simulink model "Wireless_charging"  (R2024a)
settings: Solver=VariableStepAuto  StartTime=0.0  StopTime=1  RelTol=1e-3
undefined symbols (not defined in the file): Ion, Lithium
libraries: spsSeriesRLCBranchLib x5, spsDiodeLib x4, spsMultimeterLib x4, spsIGBTDiodeLib x4, spsMeanLib x4, spsCurrentMeasurementLib x2, spsVoltageMeasurementLib x2, spsACVoltageSourceLib x1, spsUniversalBridgeLib x1, spsPWMGeneratorDCDCLib x1, spsBatteryLib x1, spsMutualInductanceLib x1
settings Model: Creator=User  LastModifiedBy=User

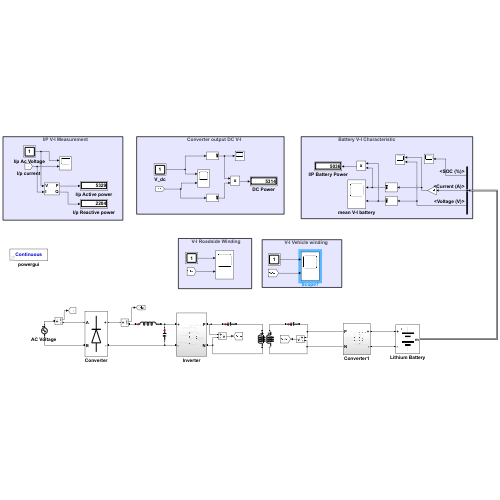
[thumbnail: Simulink's stored preview of the top-level diagram]
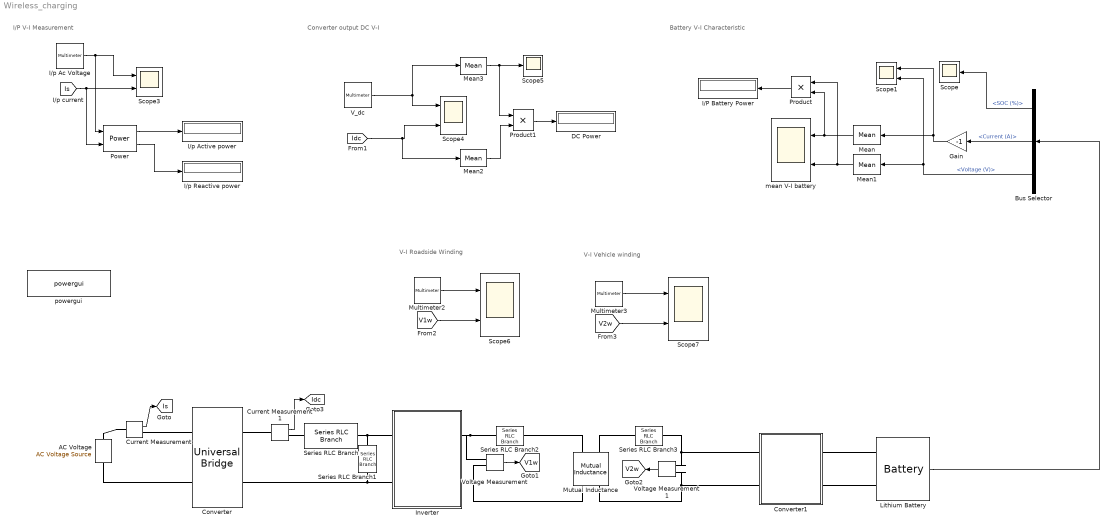
== system Wireless_charging ==
  note: V-I Roadside Winding
  note: V-I Vehicle winding
  note: Battery V-I Characteristic
  note: I/P V-I Measurement
  note: Converter output DC V-I
  "AC Voltage " : spsACVoltageSourceLib/AC Voltage Source  Amplitude=325  Phase=0  Frequency=50  SampleTime=0  Measurements=Voltage  BusType=swing  Pref=10e3  Qref=0  Qmin=-inf  Qmax=+inf
  Bus Selector : BusSelector  OutputSignals=SOC (%),Current (A),Voltage (V)
  Converter : spsUniversalBridgeLib/Universal Bridge  Arms=2  SnubberResistance=1e5  SnubberCapacitance=inf  Device=Diodes  Ron=1e-3  Lon=0  ForwardVoltages="[  0  0  ]"  ForwardVoltage=0  GTOparameters=[ 10e-6 , 20e-6 ]  IGBTparameters=[ 1e-6 , 2e-6 ]  Measurements=All voltages and currents  Measurements_2=None  converterType=Rectifier
  Converter1 : Subsystem
  Current Measurement : spsCurrentMeasurementLib/Current Measurement  PhasorSimulation=off  OutputType=Complex  PSBequivalent=0
  Current Measurement1 : spsCurrentMeasurementLib/Current Measurement  PhasorSimulation=off  OutputType=Complex  PSBequivalent=0
  DC Power : Display
  Gain : Gain  Gain=-1
  I/P Battery Power : Display
  I/p Ac Voltage : spsMultimeterLib/Multimeter  L=15  sel=8  yselected={}  Gain=1  OutputType=Complex  PlotAtSimulationStop=off  PhasorSimulation=off
  I/p Active power : Display
  I/p Reactive power : Display
  Inverter : Subsystem
  Lithium Battery : spsBatteryLib/Battery  BatType=Lithium-Ion  ShowTempParam=off  ThermalPreset=no  ShowAgeParam=off  NomV=360  NomQ=100  SOC=50  Batt_Tr=1  PresetModel=on  MaxQ=100  MinV=270  FullV=419.0354  Dis_rate=43.4783  R=0.036  Normal_OP=90.4348  expZone="[388.9389      4.913043]"  current=[6.5 13 32.5]  Units=Time  Tci=20  NomT=20  T2=-30  MaxQ2=4.8  FullV2=7.1  Normal_OP2=5.655  expZone2="[6.58           1]"  Rca=0.6  ti=2000  Dp=0  Neq0=0  Tsim=1e6  Ta1=25  Qeol=5.4*0.9  Reol=0.013333*1.2  Char_age=[2.3478, 3]  Dis_age=[2.3478, 10]  N1=1500  N2=10500  N3=1000  N4=1400  Ta2=45  N5=950
  Mean{,1..3} (4 alike) : spsMeanLib/Mean  Freq=50  Vinit=0  Ts=0
  Multimeter2 : spsMultimeterLib/Multimeter  L=15  sel=10  yselected={}  Gain=1  OutputType=Complex  PlotAtSimulationStop=off  PhasorSimulation=off
  Multimeter3 : spsMultimeterLib/Multimeter  L=15  sel=11  yselected={}  Gain=1  OutputType=Complex  PlotAtSimulationStop=off  PhasorSimulation=off
  Mutual Inductance : spsMutualInductanceLib/Mutual Inductance  LConnTagsString=a|b  RConnTagsString=A|B  TypeOfMutual=Two or three windings with equal mutual terms  NumberOfWindings=3  SelfImpedance1=[1e-3 266.16e-06]  SelfImpedance2=[ 1e-3 266.16e-06]  ThreeWindings=off  SelfImpedance3=[ 1.1 1.1e-03]  MutualImpedance=[0 85.46e-06]  InductanceMatrix="[1.0 0.9  0.9 ;  0.9 1.0  0.9;  0.9 0.9 1.0 ] * 1e-3"  ResistanceMatrix="[1.0 0.9  0.9 ;  0.9 1.0  0.9;  0.9 0.9 1.0 ]"  Measurements=None
      settings: LibrarySourceBlock=sps_lib/Passives/Mutual Inductance
  Power : spsPowerLib/Power  Freq=50  Vinit=[1, 0]  Iinit=[1, 0]  Ts=0
  Product : Product
  Product1 : Product
  Scope : Scope
  Scope{1,3..4,6..7} (5 alike) : Scope  NumInputPorts=2
  Scope5 : Scope
  Series RLC Branch : spsSeriesRLCBranchLib/Series RLC Branch  LConnTagsString=__new0  RConnTagsString=__new0  BranchType=L  Resistance=1  Inductance=10e-3  SetiL0=off  InitialCurrent=0  Capacitance=1e-6  Setx0=off  InitialVoltage=0  Measurements=Branch current
  Series RLC Branch1 : spsSeriesRLCBranchLib/Series RLC Branch  LConnTagsString=__new0  RConnTagsString=__new0  BranchType=C  Resistance=1  Inductance=1e-3  SetiL0=off  InitialCurrent=0  Capacitance=300e-6  Setx0=off  InitialVoltage=0  Measurements=None
  Series RLC Branch2 : spsSeriesRLCBranchLib/Series RLC Branch  LConnTagsString=__new0  RConnTagsString=__new0  BranchType=C  Resistance=1  Inductance=1e-3  SetiL0=off  InitialCurrent=0  Capacitance=105.74e-9  Setx0=off  InitialVoltage=0  Measurements=Branch current
  Series RLC Branch3 : spsSeriesRLCBranchLib/Series RLC Branch  LConnTagsString=__new0  RConnTagsString=__new0  BranchType=C  Resistance=1  Inductance=1e-3  SetiL0=off  InitialCurrent=0  Capacitance=109.634e-9  Setx0=off  InitialVoltage=0  Measurements=Branch current
  V_dc : spsMultimeterLib/Multimeter  L=15  sel=7  yselected={}  Gain=1  OutputType=Complex  PlotAtSimulationStop=off  PhasorSimulation=off
  Voltage Measurement : spsVoltageMeasurementLib/Voltage Measurement  PhasorSimulation=off  OutputType=Complex  PSBequivalent=0
  Voltage Measurement1 : spsVoltageMeasurementLib/Voltage Measurement  PhasorSimulation=off  OutputType=Complex  PSBequivalent=0
  mean V-I battery : Scope  NumInputPorts=2
  powergui : sps_lib/powergui  Priority=1  SimulationMode=Continuous  SampleTime=50e-6  frequency=60  Iterations=50  frequencyindice=50  Pbase=100e6  ErrMax=1e-4  UnitsV=kV  UnitsW=MW  buscounter=0  FunctionMessages=off  echomessages=off  EnableUseOfTLC=off  CurrentSourceSwitches=off  DisableSnubberDevices=off  DisableRonSwitches=off  DisableVfSwitches=off  DisplayEquations=off  AutomaticDiscreteSolvers=off  SolverType=Tustin/Backward Euler (TBE)  Interpol=off  ExternalGateDelay=off  methode=off  Ts=100  x0status=blocks  SPID=on  SwTol=0  HookPort=off  NonlinearTolerance=1e-4  nMaxIteration=100  ContinueOnMaxIteration=off  RestoreLinks=warning  ResistiveCurrentMeasurement=off  Frange=[0:2:500]  Ylog=off  Xlog=on  ShowGrid=off  save=off  variable=ZData  structure=0  ZoomFFT=off  StartTime=0.0  cycles=1  DisplayStyle=1  fundamental=60  FreqAxis=off  MaxFrequency=1000  frequencyindicesteady=1  RmsSteady=1  display=off
  tag scope: Idc=global, Is=global, V1w=global, V2w=global
  wires:
  Current Measurement/1 -> [Is]
  Voltage Measurement/1 -> [V1w]
  Voltage Measurement1/1 -> [V2w]
  Lithium Battery/1 -> Bus Selector/1
  Bus Selector/1 -> Scope/1  "<SOC (%)>"
  Bus Selector/2 -> Gain/1  "<Current (A)>"
  Gain/1 -> Mean/1, Scope1/1
  Bus Selector/3 -> Mean1/1, Scope1/2  "<Voltage (V)>"
  Mean/1 -> Product/2, mean V-I battery/1
  Mean1/1 -> Product/1, mean V-I battery/2
  Product/1 -> I/P Battery Power/1
  I/p Ac Voltage/1 -> Scope3/1, Power/1
  [Is] -> Power/2, Scope3/2
  Current Measurement1/1 -> [Idc]
  Power/2 -> I/p Reactive power/1
  Power/1 -> I/p Active power/1
  V_dc/1 -> Scope4/1, Mean3/1
  [Idc] -> Mean2/1, Scope4/2
  Mean3/1 -> Product1/1, Scope5/1
  Mean2/1 -> Product1/2
  Product1/1 -> DC Power/1
  Multimeter2/1 -> Scope6/1
  [V1w] -> Scope6/2
  Multimeter3/1 -> Scope7/1
  [V2w] -> Scope7/2
  connections:
  Current Measurement/LConn1 -- "AC Voltage "/RConn1
  Current Measurement/RConn1 -- Converter/LConn1
  Current Measurement1/LConn1 -- Converter/RConn1
  Series RLC Branch/RConn1 -- Inverter/LConn1 -- Series RLC Branch1/LConn1
  Current Measurement1/RConn1 -- Series RLC Branch/LConn1
  "AC Voltage "/LConn1 -- Converter/LConn2
  Converter/RConn2 -- Inverter/LConn2 -- Series RLC Branch1/RConn1
  Inverter/RConn1 -- Series RLC Branch2/LConn1 -- Voltage Measurement/LConn1
  Inverter/RConn2 -- Voltage Measurement/LConn2 -- Mutual Inductance/RConn1
  Series RLC Branch2/RConn1 -- Mutual Inductance/LConn1
  Series RLC Branch3/LConn1 -- Mutual Inductance/LConn2
  Voltage Measurement1/LConn1 -- Series RLC Branch3/RConn1 -- Converter1/LConn1
  Voltage Measurement1/LConn2 -- Mutual Inductance/RConn2 -- Converter1/LConn2
  Lithium Battery/LConn1 -- Converter1/RConn1
  Lithium Battery/LConn2 -- Converter1/RConn2

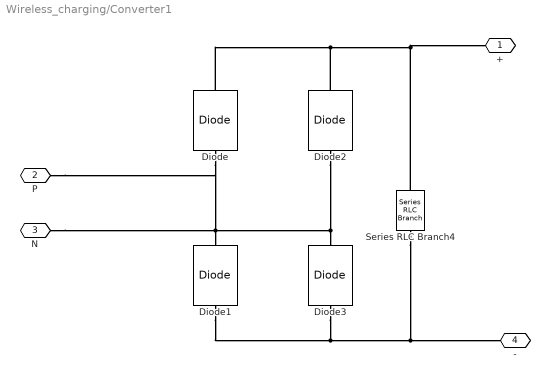
== system Wireless_charging/Converter1 ==
  Diode{,1..3} (4 alike) : spsDiodeLib/Diode  Ron=0.001  Lon=0  Vf=0.8  IC=0  UseSnubber=0  Rs=500  Cs=250e-9  Measurements=off
  Series RLC Branch4 : spsSeriesRLCBranchLib/Series RLC Branch  LConnTagsString=__new0  RConnTagsString=__new0  BranchType=C  Resistance=1  Inductance=1e-3  SetiL0=off  InitialCurrent=0  Capacitance=300e-06  Setx0=off  InitialVoltage=0  Measurements=Branch voltage
  + : PMIOPort  Side=Right
  P : PMIOPort  Port=2  Side=Left
  N : PMIOPort  Port=3  Side=Left
  - : PMIOPort  Port=4  Side=Right
  connections:
  Diode1/LConn1 -- Diode3/LConn1 -- -/RConn1 -- Series RLC Branch4/RConn1
  Diode1/RConn1 -- P/RConn1 -- Diode/LConn1
  Diode3/RConn1 -- N/RConn1 -- Diode2/LConn1
  Diode/RConn1 -- Diode2/RConn1 -- +/RConn1 -- Series RLC Branch4/LConn1

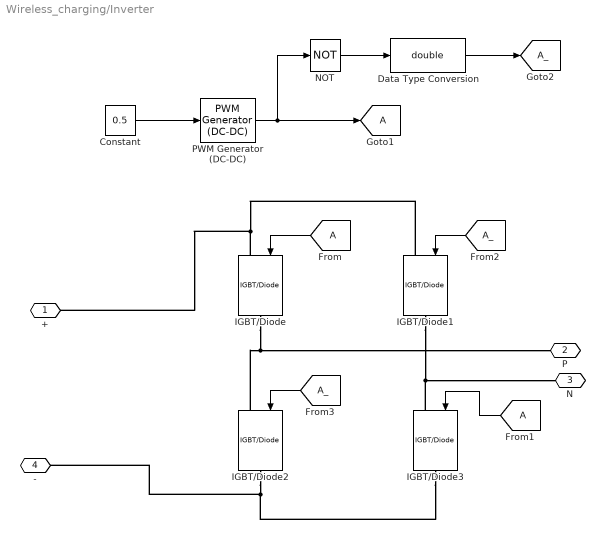
== system Wireless_charging/Inverter ==
  Constant : Constant  Value=0.5
  Data Type Conversion : DataTypeConversion  OutDataTypeStr=double  SaturateOnIntegerOverflow=off  RndMeth=Floor
  From : From  TagVisibility=global
  From1 : From  TagVisibility=global
  Goto1 : Goto  TagVisibility=global
  IGBT/Diode{,1..3} (4 alike) : spsIGBTDiodeLib/IGBT//Diode  Ron=1e-3  Rs=1e5  Cs=inf  Measurements=off
  NOT : Logic  Operator=NOT  IconShape=distinctive  AllPortsSameDT=off  OutDataTypeStr=boolean
  PWM Generator (DC-DC) : spsPWMGeneratorDCDCLib/PWM Generator (DC-DC)  Fsw=30000  Ts=0
  + : PMIOPort  Side=Left
  P : PMIOPort  Port=2  Side=Right
  N : PMIOPort  Port=3  Side=Right
  - : PMIOPort  Port=4  Side=Left
  tag scope: A_=global
  wires:
  PWM Generator (DC-DC)/1 -> Goto1/1, NOT/1
  [A_] -> IGBT/Diode2/1
  Data Type Conversion/1 -> [A_]
  Constant/1 -> PWM Generator (DC-DC)/1
  From/1 -> IGBT/Diode/1
  [A_] -> IGBT/Diode1/1
  NOT/1 -> Data Type Conversion/1
  From1/1 -> IGBT/Diode3/1
  connections:
  IGBT/Diode/LConn1 -- IGBT/Diode1/LConn1 -- +/RConn1
  IGBT/Diode3/RConn1 -- IGBT/Diode2/RConn1 -- -/RConn1
  IGBT/Diode/RConn1 -- P/RConn1 -- IGBT/Diode2/LConn1
  IGBT/Diode3/LConn1 -- IGBT/Diode1/RConn1 -- N/RConn1
